simulink model "atomic_bitches"  (Simulink 7.7)
settings: Solver=ode45  StartTime=0.0  StopTime=10.0  RelTol=1e-3
settings Model: Creator=George  LastModifiedBy=George
settings OptimizationCC: InlineParams=on

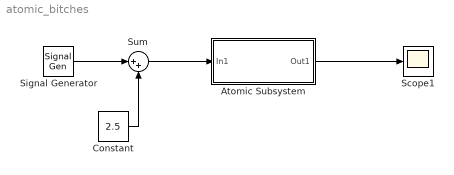
== system atomic_bitches ==
  Atomic Subsystem : Subsystem  TreatAsAtomicUnit=on
  Constant : Constant  Value=2.5
  Scope1 : Scope
      settings: TimeRange=200  YMin=1.2  YMax=3.5  SaveName=ScopeData7  MaxDataPoints=250  SampleInput=on  SampleTime=0.02
  Signal Generator : SignalGenerator  WaveForm=square  Units=rad/sec
  Sum : Sum  Inputs=|++
  wires:
  Constant/1 -> Sum/2
  Signal Generator/1 -> Sum/1
  Sum/1 -> Atomic Subsystem/1(In1)
  Atomic Subsystem/1(Out1) -> Scope1/1

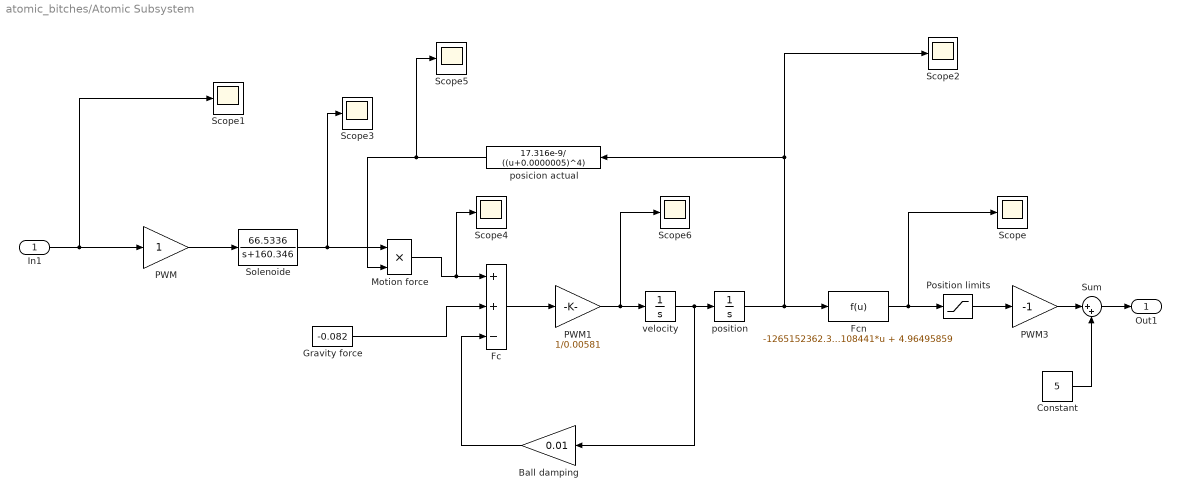
== system atomic_bitches/Atomic Subsystem ==
  In1 : Inport
  Ball damping : Gain  Gain=0.01  SaturateOnIntegerOverflow=on  OutDataTypeStr=Inherit: Same as input  ParamDataTypeStr=Inherit: Same as input
  Constant : Constant  Value=5
  Fc : Sum  Inputs=++-  SaturateOnIntegerOverflow=on  InputSameDT=on  OutDataTypeStr=Inherit: Same as first input
  Fcn : Fcn  Expr=-1265152362.37500000*u^6 + 365514542.97265600*u^5 - 37735048.55615230*u^4 + 1777017.78319550*u^3 - 37095.65220773*u^2 + 191.93108441*u + 4.96495859
  Gravity force : Constant  Value=-0.082
  Motion force : Product  SaturateOnIntegerOverflow=on  InputSameDT=on  OutDataTypeStr=Inherit: Same as first input
  PWM : Gain  SaturateOnIntegerOverflow=on  OutDataTypeStr=Inherit: Same as input  ParamDataTypeStr=Inherit: Same as input
  PWM1 : Gain  Gain=1/0.00581  SaturateOnIntegerOverflow=on  OutDataTypeStr=Inherit: Same as input  ParamDataTypeStr=Inherit: Same as input
  PWM3 : Gain  Gain=-1  SaturateOnIntegerOverflow=on  OutDataTypeStr=Inherit: Same as input  ParamDataTypeStr=Inherit: Same as input
  Position limits : Saturate  UpperLimit=5  LowerLimit=-5  ZeroCross=off
  Scope{,1..6} (7 alike) : Scope
      Scope2 settings: YMin=0.016  YMax=0.028  SaveName=ScopeData2
      Scope3 settings: YMin=0  YMax=2.25  SaveName=ScopeData3
      Scope4 settings: SaveName=ScopeData4
      Scope5 settings: YMin=0.025  YMax=0.25  SaveName=ScopeData5
      Scope6 settings: YMin=-7.5  YMax=12.5  SaveName=ScopeData6
  Solenoide : TransferFcn  Numerator=[66.5336]  Denominator=[1 160.346]
  Sum : Sum  Inputs=|++
  posicion actual : Fcn  Expr=17.316e-9/ ((u+0.0000005)^4)
  position : Integrator  LimitOutput=on  UpperSaturationLimit=0.06  LowerSaturationLimit=0  ZeroCross=off
  velocity : Integrator  UpperSaturationLimit=Inf  LowerSaturationLimit=-Inf  ZeroCross=off
  Out1 : Outport
  wires:
  PWM/1 -> Solenoide/1
  Solenoide/1 -> Motion force/1, Scope3/1
  Gravity force/1 -> Fc/2
  Motion force/1 -> Fc/1, Scope4/1
  velocity/1 -> position/1, Ball damping/1
  Ball damping/1 -> Fc/3
  posicion actual/1 -> Motion force/2, Scope5/1
  Fcn/1 -> Position limits/1, Scope/1
  In1/1 -> PWM/1, Scope1/1
  PWM1/1 -> velocity/1, Scope6/1
  Fc/1 -> PWM1/1
  Position limits/1 -> PWM3/1
  position/1 -> Fcn/1, posicion actual/1, Scope2/1
  Constant/1 -> Sum/2
  PWM3/1 -> Sum/1
  Sum/1 -> Out1/1
